simulink model "can8auto"  (R2018a)
settings: Solver=VariableStepAuto  StartTime=0.0  StopTime=5000  RelTol=1e-3
libraries: commcrc2 x20, simulink x20, simulink_extras x5, dspswit3 x5
(part 4 of 7)

== system can8auto/CAN MASTER/CAN NODE/SDO Frame generator/Subsystem/1B3 ==
  In1 : Inport
  In2 : Inport  Port=2
  In3 : Inport  Port=3
  In4 : Inport  Port=4
  Action Port : ActionPort  ActionType=case
  Mux : Mux
  Out1 : Outport
  wires:
  In4/1 -> Mux/4
  In3/1 -> Mux/3
  Mux/1 -> Out1/1
  In2/1 -> Mux/2
  In1/1 -> Mux/1

== system can8auto/CAN MASTER/CAN NODE/SDO Frame generator/Subsystem/1B4 ==
  In1 : Inport
  In2 : Inport  Port=2
  In3 : Inport  Port=3
  In4 : Inport  Port=4
  In5 : Inport  Port=5
  Action Port : ActionPort  ActionType=case
  Mux : Mux  Inputs=5
  Out1 : Outport
  wires:
  In5/1 -> Mux/5
  In4/1 -> Mux/4
  In3/1 -> Mux/3
  Mux/1 -> Out1/1
  In2/1 -> Mux/2
  In1/1 -> Mux/1

== system can8auto/CAN MASTER/CAN NODE/SDO Frame generator/Subsystem/1B5 ==
  In1 : Inport
  In2 : Inport  Port=2
  In3 : Inport  Port=3
  In4 : Inport  Port=4
  In5 : Inport  Port=5
  In6 : Inport  Port=6
  Action Port : ActionPort  ActionType=case
  Mux : Mux  Inputs=6
  Out1 : Outport
  wires:
  In6/1 -> Mux/6
  In5/1 -> Mux/5
  In4/1 -> Mux/4
  In3/1 -> Mux/3
  Mux/1 -> Out1/1
  In2/1 -> Mux/2
  In1/1 -> Mux/1

== system can8auto/CAN MASTER/CAN NODE/SDO Frame generator/Subsystem/1B6 ==
  In1 : Inport
  In2 : Inport  Port=2
  In3 : Inport  Port=3
  In4 : Inport  Port=4
  In5 : Inport  Port=5
  In6 : Inport  Port=6
  In7 : Inport  Port=7
  Action Port : ActionPort  ActionType=case
  Mux : Mux  Inputs=7
  Out1 : Outport
  wires:
  In7/1 -> Mux/7
  In6/1 -> Mux/6
  In5/1 -> Mux/5
  In4/1 -> Mux/4
  In3/1 -> Mux/3
  Mux/1 -> Out1/1
  In2/1 -> Mux/2
  In1/1 -> Mux/1

== system can8auto/CAN MASTER/CAN NODE/SDO Frame generator/Subsystem/1B7 ==
  In1 : Inport
  In2 : Inport  Port=2
  In3 : Inport  Port=3
  In4 : Inport  Port=4
  In5 : Inport  Port=5
  In6 : Inport  Port=6
  In7 : Inport  Port=7
  In8 : Inport  Port=8
  Action Port : ActionPort  ActionType=default
  Mux : Mux  Inputs=8
  Out1 : Outport
  wires:
  In8/1 -> Mux/8
  In7/1 -> Mux/7
  In6/1 -> Mux/6
  In5/1 -> Mux/5
  In4/1 -> Mux/4
  In3/1 -> Mux/3
  Mux/1 -> Out1/1
  In2/1 -> Mux/2
  In1/1 -> Mux/1

== system can8auto/CAN MASTER/CAN NODE/SDO Frame generator/Subsystem1/1B ==
  In1 : Inport
  Action Port : ActionPort  ActionType=case
  Out1 : Outport
  wires:
  In1/1 -> Out1/1

== system can8auto/CAN MASTER/CAN NODE/SDO Frame generator/Subsystem1/1B1 ==
  In1 : Inport
  In2 : Inport  Port=2
  Action Port : ActionPort  ActionType=case
  Mux : Mux  Inputs=2
  Out1 : Outport
  wires:
  Mux/1 -> Out1/1
  In2/1 -> Mux/2
  In1/1 -> Mux/1

== system can8auto/CAN MASTER/CAN NODE/SDO Frame generator/Subsystem1/1B2 ==
  In1 : Inport
  In2 : Inport  Port=2
  In3 : Inport  Port=3
  Action Port : ActionPort  ActionType=case
  Mux : Mux  Inputs=3
  Out1 : Outport
  wires:
  In3/1 -> Mux/3
  Mux/1 -> Out1/1
  In2/1 -> Mux/2
  In1/1 -> Mux/1

== system can8auto/CAN MASTER/CAN NODE/SDO Frame generator/Subsystem1/1B3 ==
  In1 : Inport
  In2 : Inport  Port=2
  In3 : Inport  Port=3
  In4 : Inport  Port=4
  Action Port : ActionPort  ActionType=case
  Mux : Mux
  Out1 : Outport
  wires:
  In4/1 -> Mux/4
  In3/1 -> Mux/3
  Mux/1 -> Out1/1
  In2/1 -> Mux/2
  In1/1 -> Mux/1

== system can8auto/CAN MASTER/CAN NODE/SDO Frame generator/Subsystem1/1B4 ==
  In1 : Inport
  In2 : Inport  Port=2
  In3 : Inport  Port=3
  In4 : Inport  Port=4
  In5 : Inport  Port=5
  Action Port : ActionPort  ActionType=case
  Mux : Mux  Inputs=5
  Out1 : Outport
  wires:
  In5/1 -> Mux/5
  In4/1 -> Mux/4
  In3/1 -> Mux/3
  Mux/1 -> Out1/1
  In2/1 -> Mux/2
  In1/1 -> Mux/1

== system can8auto/CAN MASTER/CAN NODE/SDO Frame generator/Subsystem1/1B5 ==
  In1 : Inport
  In2 : Inport  Port=2
  In3 : Inport  Port=3
  In4 : Inport  Port=4
  In5 : Inport  Port=5
  In6 : Inport  Port=6
  Action Port : ActionPort  ActionType=case
  Mux : Mux  Inputs=6
  Out1 : Outport
  wires:
  In6/1 -> Mux/6
  In5/1 -> Mux/5
  In4/1 -> Mux/4
  In3/1 -> Mux/3
  Mux/1 -> Out1/1
  In2/1 -> Mux/2
  In1/1 -> Mux/1

== system can8auto/CAN MASTER/CAN NODE/SDO Frame generator/Subsystem1/1B6 ==
  In1 : Inport
  In2 : Inport  Port=2
  In3 : Inport  Port=3
  In4 : Inport  Port=4
  In5 : Inport  Port=5
  In6 : Inport  Port=6
  In7 : Inport  Port=7
  Action Port : ActionPort  ActionType=case
  Mux : Mux  Inputs=7
  Out1 : Outport
  wires:
  In7/1 -> Mux/7
  In6/1 -> Mux/6
  In5/1 -> Mux/5
  In4/1 -> Mux/4
  In3/1 -> Mux/3
  Mux/1 -> Out1/1
  In2/1 -> Mux/2
  In1/1 -> Mux/1

== system can8auto/CAN MASTER/CAN NODE/SDO Frame generator/Subsystem1/1B7 ==
  In1 : Inport
  In2 : Inport  Port=2
  In3 : Inport  Port=3
  In4 : Inport  Port=4
  In5 : Inport  Port=5
  In6 : Inport  Port=6
  In7 : Inport  Port=7
  In8 : Inport  Port=8
  Action Port : ActionPort  ActionType=default
  Mux : Mux  Inputs=8
  Out1 : Outport
  wires:
  In8/1 -> Mux/8
  In7/1 -> Mux/7
  In6/1 -> Mux/6
  In5/1 -> Mux/5
  In4/1 -> Mux/4
  In3/1 -> Mux/3
  Mux/1 -> Out1/1
  In2/1 -> Mux/2
  In1/1 -> Mux/1

== system can8auto/CAN MASTER/CAN NODE/SDO Frame generator/Subsystem2/1B ==
  In1 : Inport
  Action Port : ActionPort  ActionType=case
  Out1 : Outport
  wires:
  In1/1 -> Out1/1

== system can8auto/CAN MASTER/CAN NODE/SDO Frame generator/Subsystem2/1B1 ==
  In1 : Inport
  In2 : Inport  Port=2
  Action Port : ActionPort  ActionType=case
  Mux : Mux  Inputs=2
  Out1 : Outport
  wires:
  Mux/1 -> Out1/1
  In2/1 -> Mux/2
  In1/1 -> Mux/1

== system can8auto/CAN MASTER/CAN NODE/SDO Frame generator/Subsystem2/1B2 ==
  In1 : Inport
  In2 : Inport  Port=2
  In3 : Inport  Port=3
  Action Port : ActionPort  ActionType=case
  Mux : Mux  Inputs=3
  Out1 : Outport
  wires:
  In3/1 -> Mux/3
  Mux/1 -> Out1/1
  In2/1 -> Mux/2
  In1/1 -> Mux/1

== system can8auto/CAN MASTER/CAN NODE/SDO Frame generator/Subsystem2/1B3 ==
  In1 : Inport
  In2 : Inport  Port=2
  In3 : Inport  Port=3
  In4 : Inport  Port=4
  Action Port : ActionPort  ActionType=case
  Mux : Mux
  Out1 : Outport
  wires:
  In4/1 -> Mux/4
  In3/1 -> Mux/3
  Mux/1 -> Out1/1
  In2/1 -> Mux/2
  In1/1 -> Mux/1

== system can8auto/CAN MASTER/CAN NODE/SDO Frame generator/Subsystem2/1B4 ==
  In1 : Inport
  In2 : Inport  Port=2
  In3 : Inport  Port=3
  In4 : Inport  Port=4
  In5 : Inport  Port=5
  Action Port : ActionPort  ActionType=case
  Mux : Mux  Inputs=5
  Out1 : Outport
  wires:
  In5/1 -> Mux/5
  In4/1 -> Mux/4
  In3/1 -> Mux/3
  Mux/1 -> Out1/1
  In2/1 -> Mux/2
  In1/1 -> Mux/1

== system can8auto/CAN MASTER/CAN NODE/SDO Frame generator/Subsystem2/1B5 ==
  In1 : Inport
  In2 : Inport  Port=2
  In3 : Inport  Port=3
  In4 : Inport  Port=4
  In5 : Inport  Port=5
  In6 : Inport  Port=6
  Action Port : ActionPort  ActionType=case
  Mux : Mux  Inputs=6
  Out1 : Outport
  wires:
  In6/1 -> Mux/6
  In5/1 -> Mux/5
  In4/1 -> Mux/4
  In3/1 -> Mux/3
  Mux/1 -> Out1/1
  In2/1 -> Mux/2
  In1/1 -> Mux/1

== system can8auto/CAN MASTER/CAN NODE/SDO Frame generator/Subsystem2/1B6 ==
  In1 : Inport
  In2 : Inport  Port=2
  In3 : Inport  Port=3
  In4 : Inport  Port=4
  In5 : Inport  Port=5
  In6 : Inport  Port=6
  In7 : Inport  Port=7
  Action Port : ActionPort  ActionType=case
  Mux : Mux  Inputs=7
  Out1 : Outport
  wires:
  In7/1 -> Mux/7
  In6/1 -> Mux/6
  In5/1 -> Mux/5
  In4/1 -> Mux/4
  In3/1 -> Mux/3
  Mux/1 -> Out1/1
  In2/1 -> Mux/2
  In1/1 -> Mux/1

== system can8auto/CAN MASTER/CAN NODE/SDO Frame generator/Subsystem2/1B7 ==
  In1 : Inport
  In2 : Inport  Port=2
  In3 : Inport  Port=3
  In4 : Inport  Port=4
  In5 : Inport  Port=5
  In6 : Inport  Port=6
  In7 : Inport  Port=7
  In8 : Inport  Port=8
  Action Port : ActionPort  ActionType=default
  Mux : Mux  Inputs=8
  Out1 : Outport
  wires:
  In8/1 -> Mux/8
  In7/1 -> Mux/7
  In6/1 -> Mux/6
  In5/1 -> Mux/5
  In4/1 -> Mux/4
  In3/1 -> Mux/3
  Mux/1 -> Out1/1
  In2/1 -> Mux/2
  In1/1 -> Mux/1

== system can8auto/CAN MASTER/CAN NODE/SDO Frame generator/Subsystem3/1B ==
  In1 : Inport
  Action Port : ActionPort  ActionType=case
  Out1 : Outport
  wires:
  In1/1 -> Out1/1

== system can8auto/CAN MASTER/CAN NODE/SDO Frame generator/Subsystem3/1B1 ==
  In1 : Inport
  In2 : Inport  Port=2
  Action Port : ActionPort  ActionType=case
  Mux : Mux  Inputs=2
  Out1 : Outport
  wires:
  Mux/1 -> Out1/1
  In2/1 -> Mux/2
  In1/1 -> Mux/1

== system can8auto/CAN MASTER/CAN NODE/SDO Frame generator/Subsystem3/1B2 ==
  In1 : Inport
  In2 : Inport  Port=2
  In3 : Inport  Port=3
  Action Port : ActionPort  ActionType=case
  Mux : Mux  Inputs=3
  Out1 : Outport
  wires:
  In3/1 -> Mux/3
  Mux/1 -> Out1/1
  In2/1 -> Mux/2
  In1/1 -> Mux/1

== system can8auto/CAN MASTER/CAN NODE/SDO Frame generator/Subsystem3/1B3 ==
  In1 : Inport
  In2 : Inport  Port=2
  In3 : Inport  Port=3
  In4 : Inport  Port=4
  Action Port : ActionPort  ActionType=case
  Mux : Mux
  Out1 : Outport
  wires:
  In4/1 -> Mux/4
  In3/1 -> Mux/3
  Mux/1 -> Out1/1
  In2/1 -> Mux/2
  In1/1 -> Mux/1

== system can8auto/CAN MASTER/CAN NODE/SDO Frame generator/Subsystem3/1B4 ==
  In1 : Inport
  In2 : Inport  Port=2
  In3 : Inport  Port=3
  In4 : Inport  Port=4
  In5 : Inport  Port=5
  Action Port : ActionPort  ActionType=case
  Mux : Mux  Inputs=5
  Out1 : Outport
  wires:
  In5/1 -> Mux/5
  In4/1 -> Mux/4
  In3/1 -> Mux/3
  Mux/1 -> Out1/1
  In2/1 -> Mux/2
  In1/1 -> Mux/1

== system can8auto/CAN MASTER/CAN NODE/SDO Frame generator/Subsystem3/1B5 ==
  In1 : Inport
  In2 : Inport  Port=2
  In3 : Inport  Port=3
  In4 : Inport  Port=4
  In5 : Inport  Port=5
  In6 : Inport  Port=6
  Action Port : ActionPort  ActionType=case
  Mux : Mux  Inputs=6
  Out1 : Outport
  wires:
  In6/1 -> Mux/6
  In5/1 -> Mux/5
  In4/1 -> Mux/4
  In3/1 -> Mux/3
  Mux/1 -> Out1/1
  In2/1 -> Mux/2
  In1/1 -> Mux/1

== system can8auto/CAN MASTER/CAN NODE/SDO Frame generator/Subsystem3/1B6 ==
  In1 : Inport
  In2 : Inport  Port=2
  In3 : Inport  Port=3
  In4 : Inport  Port=4
  In5 : Inport  Port=5
  In6 : Inport  Port=6
  In7 : Inport  Port=7
  Action Port : ActionPort  ActionType=case
  Mux : Mux  Inputs=7
  Out1 : Outport
  wires:
  In7/1 -> Mux/7
  In6/1 -> Mux/6
  In5/1 -> Mux/5
  In4/1 -> Mux/4
  In3/1 -> Mux/3
  Mux/1 -> Out1/1
  In2/1 -> Mux/2
  In1/1 -> Mux/1

== system can8auto/CAN MASTER/CAN NODE/SDO Frame generator/Subsystem3/1B7 ==
  In1 : Inport
  In2 : Inport  Port=2
  In3 : Inport  Port=3
  In4 : Inport  Port=4
  In5 : Inport  Port=5
  In6 : Inport  Port=6
  In7 : Inport  Port=7
  In8 : Inport  Port=8
  Action Port : ActionPort  ActionType=default
  Mux : Mux  Inputs=8
  Out1 : Outport
  wires:
  In8/1 -> Mux/8
  In7/1 -> Mux/7
  In6/1 -> Mux/6
  In5/1 -> Mux/5
  In4/1 -> Mux/4
  In3/1 -> Mux/3
  Mux/1 -> Out1/1
  In2/1 -> Mux/2
  In1/1 -> Mux/1

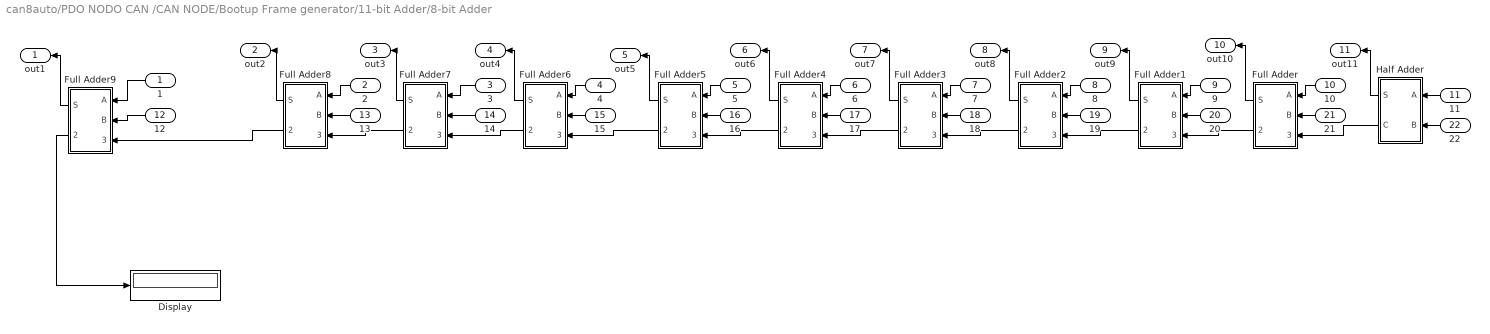
== system can8auto/PDO NODO CAN /CAN NODE/Bootup Frame generator/11-bit Adder/8-bit Adder ==
  1 : Inport
  2 : Inport  Port=2
  3 : Inport  Port=3
  4 : Inport  Port=4
  5 : Inport  Port=5
  6 : Inport  Port=6
  7 : Inport  Port=7
  8 : Inport  Port=8
  9 : Inport  Port=9
  10 : Inport  Port=10
  11 : Inport  Port=11
  12 : Inport  Port=12
  13 : Inport  Port=13
  14 : Inport  Port=14
  15 : Inport  Port=15
  16 : Inport  Port=16
  17 : Inport  Port=17
  18 : Inport  Port=18
  19 : Inport  Port=19
  20 : Inport  Port=20
  21 : Inport  Port=21
  22 : Inport  Port=22
  Display : Display
  Full Adder : Subsystem
  Full Adder1 : Subsystem
  Full Adder2 : Subsystem
  Full Adder3 : Subsystem
  Full Adder4 : Subsystem
  Full Adder5 : Subsystem
  Full Adder6 : Subsystem
  Full Adder7 : Subsystem
  Full Adder8 : Subsystem
  Full Adder9 : Subsystem
  Half Adder : Subsystem
  out1 : Outport
  out2 : Outport  Port=2
  out3 : Outport  Port=3
  out4 : Outport  Port=4
  out5 : Outport  Port=5
  out6 : Outport  Port=6
  out7 : Outport  Port=7
  out8 : Outport  Port=8
  out9 : Outport  Port=9
  out10 : Outport  Port=10
  out11 : Outport  Port=11
  wires:
  Full Adder9/2(Cout) -> Display/1
  1/1 -> Full Adder9/1(A)
  12/1 -> Full Adder9/2(B)
  13/1 -> Full Adder8/2(B)
  2/1 -> Full Adder8/1(A)
  14/1 -> Full Adder7/2(B)
  3/1 -> Full Adder7/1(A)
  Full Adder8/2(Cout) -> Full Adder9/3(Cin)
  Full Adder7/2(Cout) -> Full Adder8/3(Cin)
  Full Adder9/1(S) -> out1/1
  Full Adder8/1(S) -> out2/1
  Full Adder7/1(S) -> out3/1
  Full Adder6/2(Cout) -> Full Adder7/3(Cin)
  Half Adder/1(S) -> out11/1
  Full Adder4/1(S) -> out6/1
  Full Adder2/1(S) -> out8/1
  5/1 -> Full Adder5/1(A)
  22/1 -> Half Adder/2(B)
  Full Adder3/2(Cout) -> Full Adder4/3(Cin)
  Half Adder/2(C) -> Full Adder/3(Cin)
  Full Adder4/2(Cout) -> Full Adder5/3(Cin)
  Full Adder1/2(Cout) -> Full Adder2/3(Cin)
  Full Adder3/1(S) -> out7/1
  7/1 -> Full Adder3/1(A)
  Full Adder5/1(S) -> out5/1
  15/1 -> Full Adder6/2(B)
  19/1 -> Full Adder2/2(B)
  17/1 -> Full Adder4/2(B)
  16/1 -> Full Adder5/2(B)
  Full Adder/2(Cout) -> Full Adder1/3(Cin)
  20/1 -> Full Adder1/2(B)
  Full Adder1/1(S) -> out9/1
  6/1 -> Full Adder4/1(A)
  10/1 -> Full Adder/1(A)
  18/1 -> Full Adder3/2(B)
  4/1 -> Full Adder6/1(A)
  Full Adder6/1(S) -> out4/1
  21/1 -> Full Adder/2(B)
  Full Adder5/2(Cout) -> Full Adder6/3(Cin)
  Full Adder2/2(Cout) -> Full Adder3/3(Cin)
  11/1 -> Half Adder/1(A)
  9/1 -> Full Adder1/1(A)
  Full Adder/1(S) -> out10/1
  8/1 -> Full Adder2/1(A)

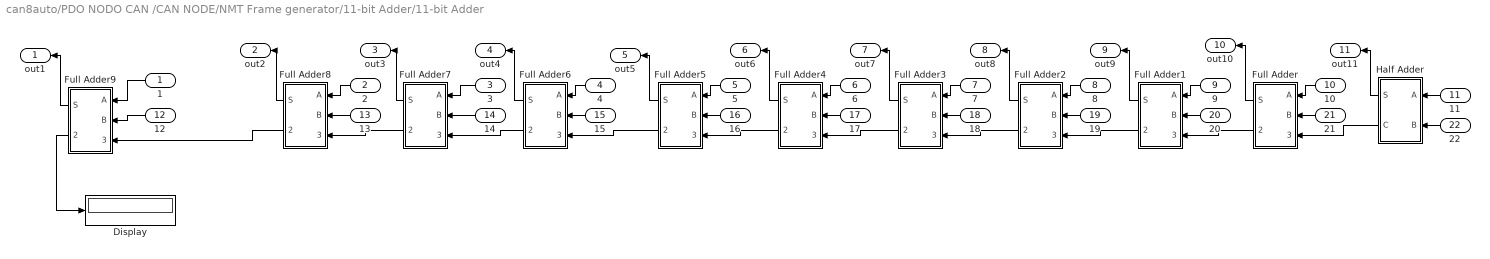
== system can8auto/PDO NODO CAN /CAN NODE/NMT Frame generator/11-bit Adder/11-bit Adder ==
  1 : Inport
  2 : Inport  Port=2
  3 : Inport  Port=3
  4 : Inport  Port=4
  5 : Inport  Port=5
  6 : Inport  Port=6
  7 : Inport  Port=7
  8 : Inport  Port=8
  9 : Inport  Port=9
  10 : Inport  Port=10
  11 : Inport  Port=11
  12 : Inport  Port=12
  13 : Inport  Port=13
  14 : Inport  Port=14
  15 : Inport  Port=15
  16 : Inport  Port=16
  17 : Inport  Port=17
  18 : Inport  Port=18
  19 : Inport  Port=19
  20 : Inport  Port=20
  21 : Inport  Port=21
  22 : Inport  Port=22
  Display : Display
  Full Adder : Subsystem
  Full Adder1 : Subsystem
  Full Adder2 : Subsystem
  Full Adder3 : Subsystem
  Full Adder4 : Subsystem
  Full Adder5 : Subsystem
  Full Adder6 : Subsystem
  Full Adder7 : Subsystem
  Full Adder8 : Subsystem
  Full Adder9 : Subsystem
  Half Adder : Subsystem
  out1 : Outport
  out2 : Outport  Port=2
  out3 : Outport  Port=3
  out4 : Outport  Port=4
  out5 : Outport  Port=5
  out6 : Outport  Port=6
  out7 : Outport  Port=7
  out8 : Outport  Port=8
  out9 : Outport  Port=9
  out10 : Outport  Port=10
  out11 : Outport  Port=11
  wires:
  Full Adder9/2(Cout) -> Display/1
  1/1 -> Full Adder9/1(A)
  12/1 -> Full Adder9/2(B)
  13/1 -> Full Adder8/2(B)
  2/1 -> Full Adder8/1(A)
  14/1 -> Full Adder7/2(B)
  3/1 -> Full Adder7/1(A)
  Full Adder8/2(Cout) -> Full Adder9/3(Cin)
  Full Adder7/2(Cout) -> Full Adder8/3(Cin)
  Full Adder9/1(S) -> out1/1
  Full Adder8/1(S) -> out2/1
  Full Adder7/1(S) -> out3/1
  Full Adder6/2(Cout) -> Full Adder7/3(Cin)
  Half Adder/1(S) -> out11/1
  Full Adder4/1(S) -> out6/1
  Full Adder2/1(S) -> out8/1
  5/1 -> Full Adder5/1(A)
  22/1 -> Half Adder/2(B)
  Full Adder3/2(Cout) -> Full Adder4/3(Cin)
  Half Adder/2(C) -> Full Adder/3(Cin)
  Full Adder4/2(Cout) -> Full Adder5/3(Cin)
  Full Adder1/2(Cout) -> Full Adder2/3(Cin)
  Full Adder3/1(S) -> out7/1
  7/1 -> Full Adder3/1(A)
  Full Adder5/1(S) -> out5/1
  15/1 -> Full Adder6/2(B)
  19/1 -> Full Adder2/2(B)
  17/1 -> Full Adder4/2(B)
  16/1 -> Full Adder5/2(B)
  Full Adder/2(Cout) -> Full Adder1/3(Cin)
  20/1 -> Full Adder1/2(B)
  Full Adder1/1(S) -> out9/1
  6/1 -> Full Adder4/1(A)
  10/1 -> Full Adder/1(A)
  18/1 -> Full Adder3/2(B)
  4/1 -> Full Adder6/1(A)
  Full Adder6/1(S) -> out4/1
  21/1 -> Full Adder/2(B)
  Full Adder5/2(Cout) -> Full Adder6/3(Cin)
  Full Adder2/2(Cout) -> Full Adder3/3(Cin)
  11/1 -> Half Adder/1(A)
  9/1 -> Full Adder1/1(A)
  Full Adder/1(S) -> out10/1
  8/1 -> Full Adder2/1(A)

== system can8auto/PDO NODO CAN /CAN NODE/PDO Frame Generator/Subsystem/1B ==
  In1 : Inport
  Action Port : ActionPort  ActionType=case
  Out1 : Outport
  wires:
  In1/1 -> Out1/1

== system can8auto/PDO NODO CAN /CAN NODE/PDO Frame Generator/Subsystem/1B1 ==
  In1 : Inport
  In2 : Inport  Port=2
  Action Port : ActionPort  ActionType=case
  Mux : Mux  Inputs=2
  Out1 : Outport
  wires:
  Mux/1 -> Out1/1
  In2/1 -> Mux/2
  In1/1 -> Mux/1

== system can8auto/PDO NODO CAN /CAN NODE/PDO Frame Generator/Subsystem/1B2 ==
  In1 : Inport
  In2 : Inport  Port=2
  In3 : Inport  Port=3
  Action Port : ActionPort  ActionType=case
  Mux : Mux  Inputs=3
  Out1 : Outport
  wires:
  In3/1 -> Mux/3
  Mux/1 -> Out1/1
  In2/1 -> Mux/2
  In1/1 -> Mux/1

== system can8auto/PDO NODO CAN /CAN NODE/PDO Frame Generator/Subsystem/1B3 ==
  In1 : Inport
  In2 : Inport  Port=2
  In3 : Inport  Port=3
  In4 : Inport  Port=4
  Action Port : ActionPort  ActionType=case
  Mux : Mux
  Out1 : Outport
  wires:
  In4/1 -> Mux/4
  In3/1 -> Mux/3
  Mux/1 -> Out1/1
  In2/1 -> Mux/2
  In1/1 -> Mux/1

== system can8auto/PDO NODO CAN /CAN NODE/PDO Frame Generator/Subsystem/1B4 ==
  In1 : Inport
  In2 : Inport  Port=2
  In3 : Inport  Port=3
  In4 : Inport  Port=4
  In5 : Inport  Port=5
  Action Port : ActionPort  ActionType=case
  Mux : Mux  Inputs=5
  Out1 : Outport
  wires:
  In5/1 -> Mux/5
  In4/1 -> Mux/4
  In3/1 -> Mux/3
  Mux/1 -> Out1/1
  In2/1 -> Mux/2
  In1/1 -> Mux/1

== system can8auto/PDO NODO CAN /CAN NODE/PDO Frame Generator/Subsystem/1B5 ==
  In1 : Inport
  In2 : Inport  Port=2
  In3 : Inport  Port=3
  In4 : Inport  Port=4
  In5 : Inport  Port=5
  In6 : Inport  Port=6
  Action Port : ActionPort  ActionType=case
  Mux : Mux  Inputs=6
  Out1 : Outport
  wires:
  In6/1 -> Mux/6
  In5/1 -> Mux/5
  In4/1 -> Mux/4
  In3/1 -> Mux/3
  Mux/1 -> Out1/1
  In2/1 -> Mux/2
  In1/1 -> Mux/1

== system can8auto/PDO NODO CAN /CAN NODE/PDO Frame Generator/Subsystem/1B6 ==
  In1 : Inport
  In2 : Inport  Port=2
  In3 : Inport  Port=3
  In4 : Inport  Port=4
  In5 : Inport  Port=5
  In6 : Inport  Port=6
  In7 : Inport  Port=7
  Action Port : ActionPort  ActionType=case
  Mux : Mux  Inputs=7
  Out1 : Outport
  wires:
  In7/1 -> Mux/7
  In6/1 -> Mux/6
  In5/1 -> Mux/5
  In4/1 -> Mux/4
  In3/1 -> Mux/3
  Mux/1 -> Out1/1
  In2/1 -> Mux/2
  In1/1 -> Mux/1

== system can8auto/PDO NODO CAN /CAN NODE/PDO Frame Generator/Subsystem/1B7 ==
  In1 : Inport
  In2 : Inport  Port=2
  In3 : Inport  Port=3
  In4 : Inport  Port=4
  In5 : Inport  Port=5
  In6 : Inport  Port=6
  In7 : Inport  Port=7
  In8 : Inport  Port=8
  Action Port : ActionPort  ActionType=default
  Mux : Mux  Inputs=8
  Out1 : Outport
  wires:
  In8/1 -> Mux/8
  In7/1 -> Mux/7
  In6/1 -> Mux/6
  In5/1 -> Mux/5
  In4/1 -> Mux/4
  In3/1 -> Mux/3
  Mux/1 -> Out1/1
  In2/1 -> Mux/2
  In1/1 -> Mux/1

== system can8auto/PDO NODO CAN /CAN NODE/SDO Frame generator/Subsystem/1B ==
  In1 : Inport
  Action Port : ActionPort  ActionType=case
  Out1 : Outport
  wires:
  In1/1 -> Out1/1

== system can8auto/PDO NODO CAN /CAN NODE/SDO Frame generator/Subsystem/1B1 ==
  In1 : Inport
  In2 : Inport  Port=2
  Action Port : ActionPort  ActionType=case
  Mux : Mux  Inputs=2
  Out1 : Outport
  wires:
  Mux/1 -> Out1/1
  In2/1 -> Mux/2
  In1/1 -> Mux/1

== system can8auto/PDO NODO CAN /CAN NODE/SDO Frame generator/Subsystem/1B2 ==
  In1 : Inport
  In2 : Inport  Port=2
  In3 : Inport  Port=3
  Action Port : ActionPort  ActionType=case
  Mux : Mux  Inputs=3
  Out1 : Outport
  wires:
  In3/1 -> Mux/3
  Mux/1 -> Out1/1
  In2/1 -> Mux/2
  In1/1 -> Mux/1

== system can8auto/PDO NODO CAN /CAN NODE/SDO Frame generator/Subsystem/1B3 ==
  In1 : Inport
  In2 : Inport  Port=2
  In3 : Inport  Port=3
  In4 : Inport  Port=4
  Action Port : ActionPort  ActionType=case
  Mux : Mux
  Out1 : Outport
  wires:
  In4/1 -> Mux/4
  In3/1 -> Mux/3
  Mux/1 -> Out1/1
  In2/1 -> Mux/2
  In1/1 -> Mux/1

== system can8auto/PDO NODO CAN /CAN NODE/SDO Frame generator/Subsystem/1B4 ==
  In1 : Inport
  In2 : Inport  Port=2
  In3 : Inport  Port=3
  In4 : Inport  Port=4
  In5 : Inport  Port=5
  Action Port : ActionPort  ActionType=case
  Mux : Mux  Inputs=5
  Out1 : Outport
  wires:
  In5/1 -> Mux/5
  In4/1 -> Mux/4
  In3/1 -> Mux/3
  Mux/1 -> Out1/1
  In2/1 -> Mux/2
  In1/1 -> Mux/1

== system can8auto/PDO NODO CAN /CAN NODE/SDO Frame generator/Subsystem/1B5 ==
  In1 : Inport
  In2 : Inport  Port=2
  In3 : Inport  Port=3
  In4 : Inport  Port=4
  In5 : Inport  Port=5
  In6 : Inport  Port=6
  Action Port : ActionPort  ActionType=case
  Mux : Mux  Inputs=6
  Out1 : Outport
  wires:
  In6/1 -> Mux/6
  In5/1 -> Mux/5
  In4/1 -> Mux/4
  In3/1 -> Mux/3
  Mux/1 -> Out1/1
  In2/1 -> Mux/2
  In1/1 -> Mux/1

== system can8auto/PDO NODO CAN /CAN NODE/SDO Frame generator/Subsystem/1B6 ==
  In1 : Inport
  In2 : Inport  Port=2
  In3 : Inport  Port=3
  In4 : Inport  Port=4
  In5 : Inport  Port=5
  In6 : Inport  Port=6
  In7 : Inport  Port=7
  Action Port : ActionPort  ActionType=case
  Mux : Mux  Inputs=7
  Out1 : Outport
  wires:
  In7/1 -> Mux/7
  In6/1 -> Mux/6
  In5/1 -> Mux/5
  In4/1 -> Mux/4
  In3/1 -> Mux/3
  Mux/1 -> Out1/1
  In2/1 -> Mux/2
  In1/1 -> Mux/1

== system can8auto/PDO NODO CAN /CAN NODE/SDO Frame generator/Subsystem/1B7 ==
  In1 : Inport
  In2 : Inport  Port=2
  In3 : Inport  Port=3
  In4 : Inport  Port=4
  In5 : Inport  Port=5
  In6 : Inport  Port=6
  In7 : Inport  Port=7
  In8 : Inport  Port=8
  Action Port : ActionPort  ActionType=default
  Mux : Mux  Inputs=8
  Out1 : Outport
  wires:
  In8/1 -> Mux/8
  In7/1 -> Mux/7
  In6/1 -> Mux/6
  In5/1 -> Mux/5
  In4/1 -> Mux/4
  In3/1 -> Mux/3
  Mux/1 -> Out1/1
  In2/1 -> Mux/2
  In1/1 -> Mux/1

== system can8auto/PDO NODO CAN /CAN NODE/SDO Frame generator/Subsystem1/1B ==
  In1 : Inport
  Action Port : ActionPort  ActionType=case
  Out1 : Outport
  wires:
  In1/1 -> Out1/1

== system can8auto/PDO NODO CAN /CAN NODE/SDO Frame generator/Subsystem1/1B1 ==
  In1 : Inport
  In2 : Inport  Port=2
  Action Port : ActionPort  ActionType=case
  Mux : Mux  Inputs=2
  Out1 : Outport
  wires:
  Mux/1 -> Out1/1
  In2/1 -> Mux/2
  In1/1 -> Mux/1

== system can8auto/PDO NODO CAN /CAN NODE/SDO Frame generator/Subsystem1/1B2 ==
  In1 : Inport
  In2 : Inport  Port=2
  In3 : Inport  Port=3
  Action Port : ActionPort  ActionType=case
  Mux : Mux  Inputs=3
  Out1 : Outport
  wires:
  In3/1 -> Mux/3
  Mux/1 -> Out1/1
  In2/1 -> Mux/2
  In1/1 -> Mux/1

== system can8auto/PDO NODO CAN /CAN NODE/SDO Frame generator/Subsystem1/1B3 ==
  In1 : Inport
  In2 : Inport  Port=2
  In3 : Inport  Port=3
  In4 : Inport  Port=4
  Action Port : ActionPort  ActionType=case
  Mux : Mux
  Out1 : Outport
  wires:
  In4/1 -> Mux/4
  In3/1 -> Mux/3
  Mux/1 -> Out1/1
  In2/1 -> Mux/2
  In1/1 -> Mux/1

== system can8auto/PDO NODO CAN /CAN NODE/SDO Frame generator/Subsystem1/1B4 ==
  In1 : Inport
  In2 : Inport  Port=2
  In3 : Inport  Port=3
  In4 : Inport  Port=4
  In5 : Inport  Port=5
  Action Port : ActionPort  ActionType=case
  Mux : Mux  Inputs=5
  Out1 : Outport
  wires:
  In5/1 -> Mux/5
  In4/1 -> Mux/4
  In3/1 -> Mux/3
  Mux/1 -> Out1/1
  In2/1 -> Mux/2
  In1/1 -> Mux/1

== system can8auto/PDO NODO CAN /CAN NODE/SDO Frame generator/Subsystem1/1B5 ==
  In1 : Inport
  In2 : Inport  Port=2
  In3 : Inport  Port=3
  In4 : Inport  Port=4
  In5 : Inport  Port=5
  In6 : Inport  Port=6
  Action Port : ActionPort  ActionType=case
  Mux : Mux  Inputs=6
  Out1 : Outport
  wires:
  In6/1 -> Mux/6
  In5/1 -> Mux/5
  In4/1 -> Mux/4
  In3/1 -> Mux/3
  Mux/1 -> Out1/1
  In2/1 -> Mux/2
  In1/1 -> Mux/1

== system can8auto/PDO NODO CAN /CAN NODE/SDO Frame generator/Subsystem1/1B6 ==
  In1 : Inport
  In2 : Inport  Port=2
  In3 : Inport  Port=3
  In4 : Inport  Port=4
  In5 : Inport  Port=5
  In6 : Inport  Port=6
  In7 : Inport  Port=7
  Action Port : ActionPort  ActionType=case
  Mux : Mux  Inputs=7
  Out1 : Outport
  wires:
  In7/1 -> Mux/7
  In6/1 -> Mux/6
  In5/1 -> Mux/5
  In4/1 -> Mux/4
  In3/1 -> Mux/3
  Mux/1 -> Out1/1
  In2/1 -> Mux/2
  In1/1 -> Mux/1

== system can8auto/PDO NODO CAN /CAN NODE/SDO Frame generator/Subsystem1/1B7 ==
  In1 : Inport
  In2 : Inport  Port=2
  In3 : Inport  Port=3
  In4 : Inport  Port=4
  In5 : Inport  Port=5
  In6 : Inport  Port=6
  In7 : Inport  Port=7
  In8 : Inport  Port=8
  Action Port : ActionPort  ActionType=default
  Mux : Mux  Inputs=8
  Out1 : Outport
  wires:
  In8/1 -> Mux/8
  In7/1 -> Mux/7
  In6/1 -> Mux/6
  In5/1 -> Mux/5
  In4/1 -> Mux/4
  In3/1 -> Mux/3
  Mux/1 -> Out1/1
  In2/1 -> Mux/2
  In1/1 -> Mux/1

== system can8auto/PDO NODO CAN /CAN NODE/SDO Frame generator/Subsystem2/1B ==
  In1 : Inport
  Action Port : ActionPort  ActionType=case
  Out1 : Outport
  wires:
  In1/1 -> Out1/1

== system can8auto/PDO NODO CAN /CAN NODE/SDO Frame generator/Subsystem2/1B1 ==
  In1 : Inport
  In2 : Inport  Port=2
  Action Port : ActionPort  ActionType=case
  Mux : Mux  Inputs=2
  Out1 : Outport
  wires:
  Mux/1 -> Out1/1
  In2/1 -> Mux/2
  In1/1 -> Mux/1

== system can8auto/PDO NODO CAN /CAN NODE/SDO Frame generator/Subsystem2/1B2 ==
  In1 : Inport
  In2 : Inport  Port=2
  In3 : Inport  Port=3
  Action Port : ActionPort  ActionType=case
  Mux : Mux  Inputs=3
  Out1 : Outport
  wires:
  In3/1 -> Mux/3
  Mux/1 -> Out1/1
  In2/1 -> Mux/2
  In1/1 -> Mux/1

== system can8auto/PDO NODO CAN /CAN NODE/SDO Frame generator/Subsystem2/1B3 ==
  In1 : Inport
  In2 : Inport  Port=2
  In3 : Inport  Port=3
  In4 : Inport  Port=4
  Action Port : ActionPort  ActionType=case
  Mux : Mux
  Out1 : Outport
  wires:
  In4/1 -> Mux/4
  In3/1 -> Mux/3
  Mux/1 -> Out1/1
  In2/1 -> Mux/2
  In1/1 -> Mux/1

== system can8auto/PDO NODO CAN /CAN NODE/SDO Frame generator/Subsystem2/1B4 ==
  In1 : Inport
  In2 : Inport  Port=2
  In3 : Inport  Port=3
  In4 : Inport  Port=4
  In5 : Inport  Port=5
  Action Port : ActionPort  ActionType=case
  Mux : Mux  Inputs=5
  Out1 : Outport
  wires:
  In5/1 -> Mux/5
  In4/1 -> Mux/4
  In3/1 -> Mux/3
  Mux/1 -> Out1/1
  In2/1 -> Mux/2
  In1/1 -> Mux/1

== system can8auto/PDO NODO CAN /CAN NODE/SDO Frame generator/Subsystem2/1B5 ==
  In1 : Inport
  In2 : Inport  Port=2
  In3 : Inport  Port=3
  In4 : Inport  Port=4
  In5 : Inport  Port=5
  In6 : Inport  Port=6
  Action Port : ActionPort  ActionType=case
  Mux : Mux  Inputs=6
  Out1 : Outport
  wires:
  In6/1 -> Mux/6
  In5/1 -> Mux/5
  In4/1 -> Mux/4
  In3/1 -> Mux/3
  Mux/1 -> Out1/1
  In2/1 -> Mux/2
  In1/1 -> Mux/1

== system can8auto/PDO NODO CAN /CAN NODE/SDO Frame generator/Subsystem2/1B6 ==
  In1 : Inport
  In2 : Inport  Port=2
  In3 : Inport  Port=3
  In4 : Inport  Port=4
  In5 : Inport  Port=5
  In6 : Inport  Port=6
  In7 : Inport  Port=7
  Action Port : ActionPort  ActionType=case
  Mux : Mux  Inputs=7
  Out1 : Outport
  wires:
  In7/1 -> Mux/7
  In6/1 -> Mux/6
  In5/1 -> Mux/5
  In4/1 -> Mux/4
  In3/1 -> Mux/3
  Mux/1 -> Out1/1
  In2/1 -> Mux/2
  In1/1 -> Mux/1

== system can8auto/PDO NODO CAN /CAN NODE/SDO Frame generator/Subsystem2/1B7 ==
  In1 : Inport
  In2 : Inport  Port=2
  In3 : Inport  Port=3
  In4 : Inport  Port=4
  In5 : Inport  Port=5
  In6 : Inport  Port=6
  In7 : Inport  Port=7
  In8 : Inport  Port=8
  Action Port : ActionPort  ActionType=default
  Mux : Mux  Inputs=8
  Out1 : Outport
  wires:
  In8/1 -> Mux/8
  In7/1 -> Mux/7
  In6/1 -> Mux/6
  In5/1 -> Mux/5
  In4/1 -> Mux/4
  In3/1 -> Mux/3
  Mux/1 -> Out1/1
  In2/1 -> Mux/2
  In1/1 -> Mux/1

== system can8auto/PDO NODO CAN /CAN NODE/SDO Frame generator/Subsystem3/1B ==
  In1 : Inport
  Action Port : ActionPort  ActionType=case
  Out1 : Outport
  wires:
  In1/1 -> Out1/1

== system can8auto/PDO NODO CAN /CAN NODE/SDO Frame generator/Subsystem3/1B1 ==
  In1 : Inport
  In2 : Inport  Port=2
  Action Port : ActionPort  ActionType=case
  Mux : Mux  Inputs=2
  Out1 : Outport
  wires:
  Mux/1 -> Out1/1
  In2/1 -> Mux/2
  In1/1 -> Mux/1

== system can8auto/PDO NODO CAN /CAN NODE/SDO Frame generator/Subsystem3/1B2 ==
  In1 : Inport
  In2 : Inport  Port=2
  In3 : Inport  Port=3
  Action Port : ActionPort  ActionType=case
  Mux : Mux  Inputs=3
  Out1 : Outport
  wires:
  In3/1 -> Mux/3
  Mux/1 -> Out1/1
  In2/1 -> Mux/2
  In1/1 -> Mux/1

== system can8auto/PDO NODO CAN /CAN NODE/SDO Frame generator/Subsystem3/1B3 ==
  In1 : Inport
  In2 : Inport  Port=2
  In3 : Inport  Port=3
  In4 : Inport  Port=4
  Action Port : ActionPort  ActionType=case
  Mux : Mux
  Out1 : Outport
  wires:
  In4/1 -> Mux/4
  In3/1 -> Mux/3
  Mux/1 -> Out1/1
  In2/1 -> Mux/2
  In1/1 -> Mux/1

== system can8auto/PDO NODO CAN /CAN NODE/SDO Frame generator/Subsystem3/1B4 ==
  In1 : Inport
  In2 : Inport  Port=2
  In3 : Inport  Port=3
  In4 : Inport  Port=4
  In5 : Inport  Port=5
  Action Port : ActionPort  ActionType=case
  Mux : Mux  Inputs=5
  Out1 : Outport
  wires:
  In5/1 -> Mux/5
  In4/1 -> Mux/4
  In3/1 -> Mux/3
  Mux/1 -> Out1/1
  In2/1 -> Mux/2
  In1/1 -> Mux/1

== system can8auto/PDO NODO CAN /CAN NODE/SDO Frame generator/Subsystem3/1B5 ==
  In1 : Inport
  In2 : Inport  Port=2
  In3 : Inport  Port=3
  In4 : Inport  Port=4
  In5 : Inport  Port=5
  In6 : Inport  Port=6
  Action Port : ActionPort  ActionType=case
  Mux : Mux  Inputs=6
  Out1 : Outport
  wires:
  In6/1 -> Mux/6
  In5/1 -> Mux/5
  In4/1 -> Mux/4
  In3/1 -> Mux/3
  Mux/1 -> Out1/1
  In2/1 -> Mux/2
  In1/1 -> Mux/1

== system can8auto/PDO NODO CAN /CAN NODE/SDO Frame generator/Subsystem3/1B6 ==
  In1 : Inport
  In2 : Inport  Port=2
  In3 : Inport  Port=3
  In4 : Inport  Port=4
  In5 : Inport  Port=5
  In6 : Inport  Port=6
  In7 : Inport  Port=7
  Action Port : ActionPort  ActionType=case
  Mux : Mux  Inputs=7
  Out1 : Outport
  wires:
  In7/1 -> Mux/7
  In6/1 -> Mux/6
  In5/1 -> Mux/5
  In4/1 -> Mux/4
  In3/1 -> Mux/3
  Mux/1 -> Out1/1
  In2/1 -> Mux/2
  In1/1 -> Mux/1

== system can8auto/PDO NODO CAN /CAN NODE/SDO Frame generator/Subsystem3/1B7 ==
  In1 : Inport
  In2 : Inport  Port=2
  In3 : Inport  Port=3
  In4 : Inport  Port=4
  In5 : Inport  Port=5
  In6 : Inport  Port=6
  In7 : Inport  Port=7
  In8 : Inport  Port=8
  Action Port : ActionPort  ActionType=default
  Mux : Mux  Inputs=8
  Out1 : Outport
  wires:
  In8/1 -> Mux/8
  In7/1 -> Mux/7
  In6/1 -> Mux/6
  In5/1 -> Mux/5
  In4/1 -> Mux/4
  In3/1 -> Mux/3
  Mux/1 -> Out1/1
  In2/1 -> Mux/2
  In1/1 -> Mux/1

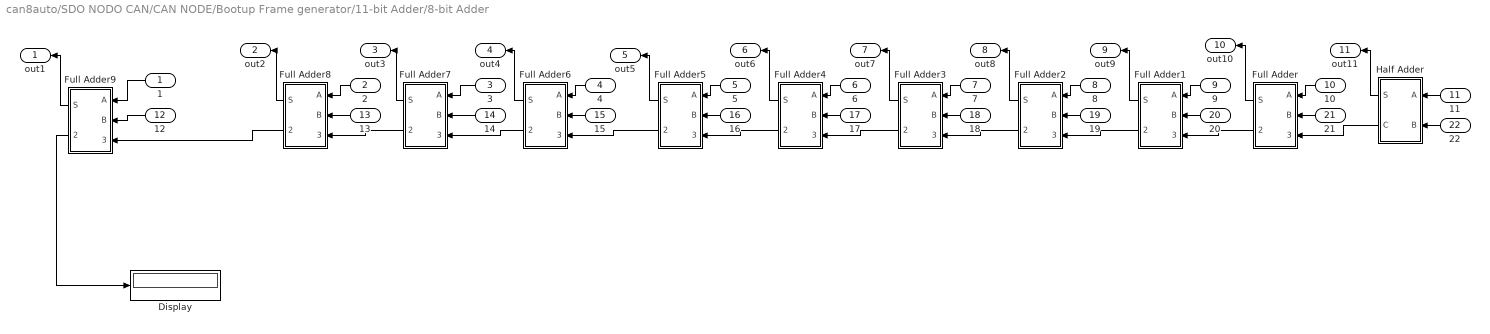
== system can8auto/SDO NODO CAN/CAN NODE/Bootup Frame generator/11-bit Adder/8-bit Adder ==
  1 : Inport
  2 : Inport  Port=2
  3 : Inport  Port=3
  4 : Inport  Port=4
  5 : Inport  Port=5
  6 : Inport  Port=6
  7 : Inport  Port=7
  8 : Inport  Port=8
  9 : Inport  Port=9
  10 : Inport  Port=10
  11 : Inport  Port=11
  12 : Inport  Port=12
  13 : Inport  Port=13
  14 : Inport  Port=14
  15 : Inport  Port=15
  16 : Inport  Port=16
  17 : Inport  Port=17
  18 : Inport  Port=18
  19 : Inport  Port=19
  20 : Inport  Port=20
  21 : Inport  Port=21
  22 : Inport  Port=22
  Display : Display
  Full Adder : Subsystem
  Full Adder1 : Subsystem
  Full Adder2 : Subsystem
  Full Adder3 : Subsystem
  Full Adder4 : Subsystem
  Full Adder5 : Subsystem
  Full Adder6 : Subsystem
  Full Adder7 : Subsystem
  Full Adder8 : Subsystem
  Full Adder9 : Subsystem
  Half Adder : Subsystem
  out1 : Outport
  out2 : Outport  Port=2
  out3 : Outport  Port=3
  out4 : Outport  Port=4
  out5 : Outport  Port=5
  out6 : Outport  Port=6
  out7 : Outport  Port=7
  out8 : Outport  Port=8
  out9 : Outport  Port=9
  out10 : Outport  Port=10
  out11 : Outport  Port=11
  wires:
  Full Adder9/2(Cout) -> Display/1
  1/1 -> Full Adder9/1(A)
  12/1 -> Full Adder9/2(B)
  13/1 -> Full Adder8/2(B)
  2/1 -> Full Adder8/1(A)
  14/1 -> Full Adder7/2(B)
  3/1 -> Full Adder7/1(A)
  Full Adder8/2(Cout) -> Full Adder9/3(Cin)
  Full Adder7/2(Cout) -> Full Adder8/3(Cin)
  Full Adder9/1(S) -> out1/1
  Full Adder8/1(S) -> out2/1
  Full Adder7/1(S) -> out3/1
  Full Adder6/2(Cout) -> Full Adder7/3(Cin)
  Half Adder/1(S) -> out11/1
  Full Adder4/1(S) -> out6/1
  Full Adder2/1(S) -> out8/1
  5/1 -> Full Adder5/1(A)
  22/1 -> Half Adder/2(B)
  Full Adder3/2(Cout) -> Full Adder4/3(Cin)
  Half Adder/2(C) -> Full Adder/3(Cin)
  Full Adder4/2(Cout) -> Full Adder5/3(Cin)
  Full Adder1/2(Cout) -> Full Adder2/3(Cin)
  Full Adder3/1(S) -> out7/1
  7/1 -> Full Adder3/1(A)
  Full Adder5/1(S) -> out5/1
  15/1 -> Full Adder6/2(B)
  19/1 -> Full Adder2/2(B)
  17/1 -> Full Adder4/2(B)
  16/1 -> Full Adder5/2(B)
  Full Adder/2(Cout) -> Full Adder1/3(Cin)
  20/1 -> Full Adder1/2(B)
  Full Adder1/1(S) -> out9/1
  6/1 -> Full Adder4/1(A)
  10/1 -> Full Adder/1(A)
  18/1 -> Full Adder3/2(B)
  4/1 -> Full Adder6/1(A)
  Full Adder6/1(S) -> out4/1
  21/1 -> Full Adder/2(B)
  Full Adder5/2(Cout) -> Full Adder6/3(Cin)
  Full Adder2/2(Cout) -> Full Adder3/3(Cin)
  11/1 -> Half Adder/1(A)
  9/1 -> Full Adder1/1(A)
  Full Adder/1(S) -> out10/1
  8/1 -> Full Adder2/1(A)

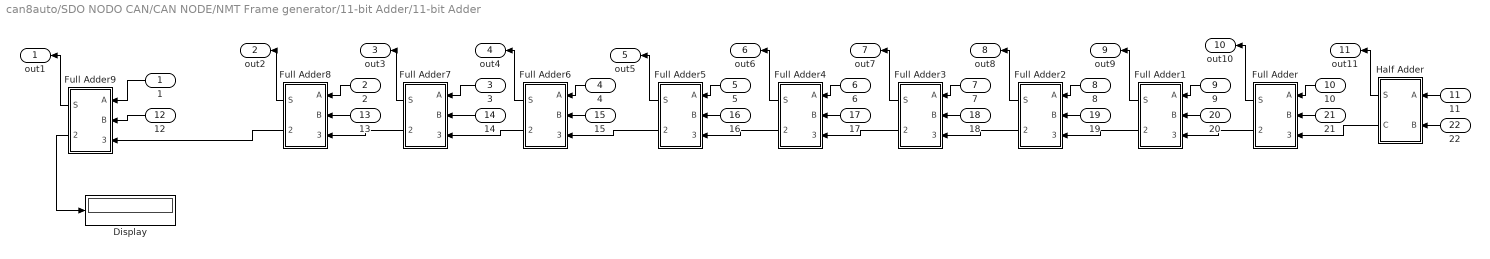
== system can8auto/SDO NODO CAN/CAN NODE/NMT Frame generator/11-bit Adder/11-bit Adder ==
  1 : Inport
  2 : Inport  Port=2
  3 : Inport  Port=3
  4 : Inport  Port=4
  5 : Inport  Port=5
  6 : Inport  Port=6
  7 : Inport  Port=7
  8 : Inport  Port=8
  9 : Inport  Port=9
  10 : Inport  Port=10
  11 : Inport  Port=11
  12 : Inport  Port=12
  13 : Inport  Port=13
  14 : Inport  Port=14
  15 : Inport  Port=15
  16 : Inport  Port=16
  17 : Inport  Port=17
  18 : Inport  Port=18
  19 : Inport  Port=19
  20 : Inport  Port=20
  21 : Inport  Port=21
  22 : Inport  Port=22
  Display : Display
  Full Adder : Subsystem
  Full Adder1 : Subsystem
  Full Adder2 : Subsystem
  Full Adder3 : Subsystem
  Full Adder4 : Subsystem
  Full Adder5 : Subsystem
  Full Adder6 : Subsystem
  Full Adder7 : Subsystem
  Full Adder8 : Subsystem
  Full Adder9 : Subsystem
  Half Adder : Subsystem
  out1 : Outport
  out2 : Outport  Port=2
  out3 : Outport  Port=3
  out4 : Outport  Port=4
  out5 : Outport  Port=5
  out6 : Outport  Port=6
  out7 : Outport  Port=7
  out8 : Outport  Port=8
  out9 : Outport  Port=9
  out10 : Outport  Port=10
  out11 : Outport  Port=11
  wires:
  Full Adder9/2(Cout) -> Display/1
  1/1 -> Full Adder9/1(A)
  12/1 -> Full Adder9/2(B)
  13/1 -> Full Adder8/2(B)
  2/1 -> Full Adder8/1(A)
  14/1 -> Full Adder7/2(B)
  3/1 -> Full Adder7/1(A)
  Full Adder8/2(Cout) -> Full Adder9/3(Cin)
  Full Adder7/2(Cout) -> Full Adder8/3(Cin)
  Full Adder9/1(S) -> out1/1
  Full Adder8/1(S) -> out2/1
  Full Adder7/1(S) -> out3/1
  Full Adder6/2(Cout) -> Full Adder7/3(Cin)
  Half Adder/1(S) -> out11/1
  Full Adder4/1(S) -> out6/1
  Full Adder2/1(S) -> out8/1
  5/1 -> Full Adder5/1(A)
  22/1 -> Half Adder/2(B)
  Full Adder3/2(Cout) -> Full Adder4/3(Cin)
  Half Adder/2(C) -> Full Adder/3(Cin)
  Full Adder4/2(Cout) -> Full Adder5/3(Cin)
  Full Adder1/2(Cout) -> Full Adder2/3(Cin)
  Full Adder3/1(S) -> out7/1
  7/1 -> Full Adder3/1(A)
  Full Adder5/1(S) -> out5/1
  15/1 -> Full Adder6/2(B)
  19/1 -> Full Adder2/2(B)
  17/1 -> Full Adder4/2(B)
  16/1 -> Full Adder5/2(B)
  Full Adder/2(Cout) -> Full Adder1/3(Cin)
  20/1 -> Full Adder1/2(B)
  Full Adder1/1(S) -> out9/1
  6/1 -> Full Adder4/1(A)
  10/1 -> Full Adder/1(A)
  18/1 -> Full Adder3/2(B)
  4/1 -> Full Adder6/1(A)
  Full Adder6/1(S) -> out4/1
  21/1 -> Full Adder/2(B)
  Full Adder5/2(Cout) -> Full Adder6/3(Cin)
  Full Adder2/2(Cout) -> Full Adder3/3(Cin)
  11/1 -> Half Adder/1(A)
  9/1 -> Full Adder1/1(A)
  Full Adder/1(S) -> out10/1
  8/1 -> Full Adder2/1(A)

== system can8auto/SDO NODO CAN/CAN NODE/PDO Frame Generator/Subsystem/1B ==
  In1 : Inport
  Action Port : ActionPort  ActionType=case
  Out1 : Outport
  wires:
  In1/1 -> Out1/1

== system can8auto/SDO NODO CAN/CAN NODE/PDO Frame Generator/Subsystem/1B1 ==
  In1 : Inport
  In2 : Inport  Port=2
  Action Port : ActionPort  ActionType=case
  Mux : Mux  Inputs=2
  Out1 : Outport
  wires:
  Mux/1 -> Out1/1
  In2/1 -> Mux/2
  In1/1 -> Mux/1

== system can8auto/SDO NODO CAN/CAN NODE/PDO Frame Generator/Subsystem/1B2 ==
  In1 : Inport
  In2 : Inport  Port=2
  In3 : Inport  Port=3
  Action Port : ActionPort  ActionType=case
  Mux : Mux  Inputs=3
  Out1 : Outport
  wires:
  In3/1 -> Mux/3
  Mux/1 -> Out1/1
  In2/1 -> Mux/2
  In1/1 -> Mux/1

== system can8auto/SDO NODO CAN/CAN NODE/PDO Frame Generator/Subsystem/1B3 ==
  In1 : Inport
  In2 : Inport  Port=2
  In3 : Inport  Port=3
  In4 : Inport  Port=4
  Action Port : ActionPort  ActionType=case
  Mux : Mux
  Out1 : Outport
  wires:
  In4/1 -> Mux/4
  In3/1 -> Mux/3
  Mux/1 -> Out1/1
  In2/1 -> Mux/2
  In1/1 -> Mux/1

== system can8auto/SDO NODO CAN/CAN NODE/PDO Frame Generator/Subsystem/1B4 ==
  In1 : Inport
  In2 : Inport  Port=2
  In3 : Inport  Port=3
  In4 : Inport  Port=4
  In5 : Inport  Port=5
  Action Port : ActionPort  ActionType=case
  Mux : Mux  Inputs=5
  Out1 : Outport
  wires:
  In5/1 -> Mux/5
  In4/1 -> Mux/4
  In3/1 -> Mux/3
  Mux/1 -> Out1/1
  In2/1 -> Mux/2
  In1/1 -> Mux/1

== system can8auto/SDO NODO CAN/CAN NODE/PDO Frame Generator/Subsystem/1B5 ==
  In1 : Inport
  In2 : Inport  Port=2
  In3 : Inport  Port=3
  In4 : Inport  Port=4
  In5 : Inport  Port=5
  In6 : Inport  Port=6
  Action Port : ActionPort  ActionType=case
  Mux : Mux  Inputs=6
  Out1 : Outport
  wires:
  In6/1 -> Mux/6
  In5/1 -> Mux/5
  In4/1 -> Mux/4
  In3/1 -> Mux/3
  Mux/1 -> Out1/1
  In2/1 -> Mux/2
  In1/1 -> Mux/1

== system can8auto/SDO NODO CAN/CAN NODE/PDO Frame Generator/Subsystem/1B6 ==
  In1 : Inport
  In2 : Inport  Port=2
  In3 : Inport  Port=3
  In4 : Inport  Port=4
  In5 : Inport  Port=5
  In6 : Inport  Port=6
  In7 : Inport  Port=7
  Action Port : ActionPort  ActionType=case
  Mux : Mux  Inputs=7
  Out1 : Outport
  wires:
  In7/1 -> Mux/7
  In6/1 -> Mux/6
  In5/1 -> Mux/5
  In4/1 -> Mux/4
  In3/1 -> Mux/3
  Mux/1 -> Out1/1
  In2/1 -> Mux/2
  In1/1 -> Mux/1

== system can8auto/SDO NODO CAN/CAN NODE/PDO Frame Generator/Subsystem/1B7 ==
  In1 : Inport
  In2 : Inport  Port=2
  In3 : Inport  Port=3
  In4 : Inport  Port=4
  In5 : Inport  Port=5
  In6 : Inport  Port=6
  In7 : Inport  Port=7
  In8 : Inport  Port=8
  Action Port : ActionPort  ActionType=default
  Mux : Mux  Inputs=8
  Out1 : Outport
  wires:
  In8/1 -> Mux/8
  In7/1 -> Mux/7
  In6/1 -> Mux/6
  In5/1 -> Mux/5
  In4/1 -> Mux/4
  In3/1 -> Mux/3
  Mux/1 -> Out1/1
  In2/1 -> Mux/2
  In1/1 -> Mux/1

== system can8auto/SDO NODO CAN/CAN NODE/SDO Frame generator/Subsystem/1B ==
  In1 : Inport
  Action Port : ActionPort  ActionType=case
  Out1 : Outport
  wires:
  In1/1 -> Out1/1

== system can8auto/SDO NODO CAN/CAN NODE/SDO Frame generator/Subsystem/1B1 ==
  In1 : Inport
  In2 : Inport  Port=2
  Action Port : ActionPort  ActionType=case
  Mux : Mux  Inputs=2
  Out1 : Outport
  wires:
  Mux/1 -> Out1/1
  In2/1 -> Mux/2
  In1/1 -> Mux/1

== system can8auto/SDO NODO CAN/CAN NODE/SDO Frame generator/Subsystem/1B2 ==
  In1 : Inport
  In2 : Inport  Port=2
  In3 : Inport  Port=3
  Action Port : ActionPort  ActionType=case
  Mux : Mux  Inputs=3
  Out1 : Outport
  wires:
  In3/1 -> Mux/3
  Mux/1 -> Out1/1
  In2/1 -> Mux/2
  In1/1 -> Mux/1

== system can8auto/SDO NODO CAN/CAN NODE/SDO Frame generator/Subsystem/1B3 ==
  In1 : Inport
  In2 : Inport  Port=2
  In3 : Inport  Port=3
  In4 : Inport  Port=4
  Action Port : ActionPort  ActionType=case
  Mux : Mux
  Out1 : Outport
  wires:
  In4/1 -> Mux/4
  In3/1 -> Mux/3
  Mux/1 -> Out1/1
  In2/1 -> Mux/2
  In1/1 -> Mux/1

== system can8auto/SDO NODO CAN/CAN NODE/SDO Frame generator/Subsystem/1B4 ==
  In1 : Inport
  In2 : Inport  Port=2
  In3 : Inport  Port=3
  In4 : Inport  Port=4
  In5 : Inport  Port=5
  Action Port : ActionPort  ActionType=case
  Mux : Mux  Inputs=5
  Out1 : Outport
  wires:
  In5/1 -> Mux/5
  In4/1 -> Mux/4
  In3/1 -> Mux/3
  Mux/1 -> Out1/1
  In2/1 -> Mux/2
  In1/1 -> Mux/1

== system can8auto/SDO NODO CAN/CAN NODE/SDO Frame generator/Subsystem/1B5 ==
  In1 : Inport
  In2 : Inport  Port=2
  In3 : Inport  Port=3
  In4 : Inport  Port=4
  In5 : Inport  Port=5
  In6 : Inport  Port=6
  Action Port : ActionPort  ActionType=case
  Mux : Mux  Inputs=6
  Out1 : Outport
  wires:
  In6/1 -> Mux/6
  In5/1 -> Mux/5
  In4/1 -> Mux/4
  In3/1 -> Mux/3
  Mux/1 -> Out1/1
  In2/1 -> Mux/2
  In1/1 -> Mux/1

== system can8auto/SDO NODO CAN/CAN NODE/SDO Frame generator/Subsystem/1B6 ==
  In1 : Inport
  In2 : Inport  Port=2
  In3 : Inport  Port=3
  In4 : Inport  Port=4
  In5 : Inport  Port=5
  In6 : Inport  Port=6
  In7 : Inport  Port=7
  Action Port : ActionPort  ActionType=case
  Mux : Mux  Inputs=7
  Out1 : Outport
  wires:
  In7/1 -> Mux/7
  In6/1 -> Mux/6
  In5/1 -> Mux/5
  In4/1 -> Mux/4
  In3/1 -> Mux/3
  Mux/1 -> Out1/1
  In2/1 -> Mux/2
  In1/1 -> Mux/1

== system can8auto/SDO NODO CAN/CAN NODE/SDO Frame generator/Subsystem/1B7 ==
  In1 : Inport
  In2 : Inport  Port=2
  In3 : Inport  Port=3
  In4 : Inport  Port=4
  In5 : Inport  Port=5
  In6 : Inport  Port=6
  In7 : Inport  Port=7
  In8 : Inport  Port=8
  Action Port : ActionPort  ActionType=default
  Mux : Mux  Inputs=8
  Out1 : Outport
  wires:
  In8/1 -> Mux/8
  In7/1 -> Mux/7
  In6/1 -> Mux/6
  In5/1 -> Mux/5
  In4/1 -> Mux/4
  In3/1 -> Mux/3
  Mux/1 -> Out1/1
  In2/1 -> Mux/2
  In1/1 -> Mux/1

== system can8auto/SDO NODO CAN/CAN NODE/SDO Frame generator/Subsystem1/1B ==
  In1 : Inport
  Action Port : ActionPort  ActionType=case
  Out1 : Outport
  wires:
  In1/1 -> Out1/1

== system can8auto/SDO NODO CAN/CAN NODE/SDO Frame generator/Subsystem1/1B1 ==
  In1 : Inport
  In2 : Inport  Port=2
  Action Port : ActionPort  ActionType=case
  Mux : Mux  Inputs=2
  Out1 : Outport
  wires:
  Mux/1 -> Out1/1
  In2/1 -> Mux/2
  In1/1 -> Mux/1

== system can8auto/SDO NODO CAN/CAN NODE/SDO Frame generator/Subsystem1/1B2 ==
  In1 : Inport
  In2 : Inport  Port=2
  In3 : Inport  Port=3
  Action Port : ActionPort  ActionType=case
  Mux : Mux  Inputs=3
  Out1 : Outport
  wires:
  In3/1 -> Mux/3
  Mux/1 -> Out1/1
  In2/1 -> Mux/2
  In1/1 -> Mux/1

== system can8auto/SDO NODO CAN/CAN NODE/SDO Frame generator/Subsystem1/1B3 ==
  In1 : Inport
  In2 : Inport  Port=2
  In3 : Inport  Port=3
  In4 : Inport  Port=4
  Action Port : ActionPort  ActionType=case
  Mux : Mux
  Out1 : Outport
  wires:
  In4/1 -> Mux/4
  In3/1 -> Mux/3
  Mux/1 -> Out1/1
  In2/1 -> Mux/2
  In1/1 -> Mux/1

== system can8auto/SDO NODO CAN/CAN NODE/SDO Frame generator/Subsystem1/1B4 ==
  In1 : Inport
  In2 : Inport  Port=2
  In3 : Inport  Port=3
  In4 : Inport  Port=4
  In5 : Inport  Port=5
  Action Port : ActionPort  ActionType=case
  Mux : Mux  Inputs=5
  Out1 : Outport
  wires:
  In5/1 -> Mux/5
  In4/1 -> Mux/4
  In3/1 -> Mux/3
  Mux/1 -> Out1/1
  In2/1 -> Mux/2
  In1/1 -> Mux/1

== system can8auto/SDO NODO CAN/CAN NODE/SDO Frame generator/Subsystem1/1B5 ==
  In1 : Inport
  In2 : Inport  Port=2
  In3 : Inport  Port=3
  In4 : Inport  Port=4
  In5 : Inport  Port=5
  In6 : Inport  Port=6
  Action Port : ActionPort  ActionType=case
  Mux : Mux  Inputs=6
  Out1 : Outport
  wires:
  In6/1 -> Mux/6
  In5/1 -> Mux/5
  In4/1 -> Mux/4
  In3/1 -> Mux/3
  Mux/1 -> Out1/1
  In2/1 -> Mux/2
  In1/1 -> Mux/1

== system can8auto/SDO NODO CAN/CAN NODE/SDO Frame generator/Subsystem1/1B6 ==
  In1 : Inport
  In2 : Inport  Port=2
  In3 : Inport  Port=3
  In4 : Inport  Port=4
  In5 : Inport  Port=5
  In6 : Inport  Port=6
  In7 : Inport  Port=7
  Action Port : ActionPort  ActionType=case
  Mux : Mux  Inputs=7
  Out1 : Outport
  wires:
  In7/1 -> Mux/7
  In6/1 -> Mux/6
  In5/1 -> Mux/5
  In4/1 -> Mux/4
  In3/1 -> Mux/3
  Mux/1 -> Out1/1
  In2/1 -> Mux/2
  In1/1 -> Mux/1

== system can8auto/SDO NODO CAN/CAN NODE/SDO Frame generator/Subsystem1/1B7 ==
  In1 : Inport
  In2 : Inport  Port=2
  In3 : Inport  Port=3
  In4 : Inport  Port=4
  In5 : Inport  Port=5
  In6 : Inport  Port=6
  In7 : Inport  Port=7
  In8 : Inport  Port=8
  Action Port : ActionPort  ActionType=default
  Mux : Mux  Inputs=8
  Out1 : Outport
  wires:
  In8/1 -> Mux/8
  In7/1 -> Mux/7
  In6/1 -> Mux/6
  In5/1 -> Mux/5
  In4/1 -> Mux/4
  In3/1 -> Mux/3
  Mux/1 -> Out1/1
  In2/1 -> Mux/2
  In1/1 -> Mux/1

== system can8auto/SDO NODO CAN/CAN NODE/SDO Frame generator/Subsystem2/1B ==
  In1 : Inport
  Action Port : ActionPort  ActionType=case
  Out1 : Outport
  wires:
  In1/1 -> Out1/1

== system can8auto/SDO NODO CAN/CAN NODE/SDO Frame generator/Subsystem2/1B1 ==
  In1 : Inport
  In2 : Inport  Port=2
  Action Port : ActionPort  ActionType=case
  Mux : Mux  Inputs=2
  Out1 : Outport
  wires:
  Mux/1 -> Out1/1
  In2/1 -> Mux/2
  In1/1 -> Mux/1

== system can8auto/SDO NODO CAN/CAN NODE/SDO Frame generator/Subsystem2/1B2 ==
  In1 : Inport
  In2 : Inport  Port=2
  In3 : Inport  Port=3
  Action Port : ActionPort  ActionType=case
  Mux : Mux  Inputs=3
  Out1 : Outport
  wires:
  In3/1 -> Mux/3
  Mux/1 -> Out1/1
  In2/1 -> Mux/2
  In1/1 -> Mux/1

== system can8auto/SDO NODO CAN/CAN NODE/SDO Frame generator/Subsystem2/1B3 ==
  In1 : Inport
  In2 : Inport  Port=2
  In3 : Inport  Port=3
  In4 : Inport  Port=4
  Action Port : ActionPort  ActionType=case
  Mux : Mux
  Out1 : Outport
  wires:
  In4/1 -> Mux/4
  In3/1 -> Mux/3
  Mux/1 -> Out1/1
  In2/1 -> Mux/2
  In1/1 -> Mux/1

== system can8auto/SDO NODO CAN/CAN NODE/SDO Frame generator/Subsystem2/1B4 ==
  In1 : Inport
  In2 : Inport  Port=2
  In3 : Inport  Port=3
  In4 : Inport  Port=4
  In5 : Inport  Port=5
  Action Port : ActionPort  ActionType=case
  Mux : Mux  Inputs=5
  Out1 : Outport
  wires:
  In5/1 -> Mux/5
  In4/1 -> Mux/4
  In3/1 -> Mux/3
  Mux/1 -> Out1/1
  In2/1 -> Mux/2
  In1/1 -> Mux/1

== system can8auto/SDO NODO CAN/CAN NODE/SDO Frame generator/Subsystem2/1B5 ==
  In1 : Inport
  In2 : Inport  Port=2
  In3 : Inport  Port=3
  In4 : Inport  Port=4
  In5 : Inport  Port=5
  In6 : Inport  Port=6
  Action Port : ActionPort  ActionType=case
  Mux : Mux  Inputs=6
  Out1 : Outport
  wires:
  In6/1 -> Mux/6
  In5/1 -> Mux/5
  In4/1 -> Mux/4
  In3/1 -> Mux/3
  Mux/1 -> Out1/1
  In2/1 -> Mux/2
  In1/1 -> Mux/1

== system can8auto/SDO NODO CAN/CAN NODE/SDO Frame generator/Subsystem2/1B6 ==
  In1 : Inport
  In2 : Inport  Port=2
  In3 : Inport  Port=3
  In4 : Inport  Port=4
  In5 : Inport  Port=5
  In6 : Inport  Port=6
  In7 : Inport  Port=7
  Action Port : ActionPort  ActionType=case
  Mux : Mux  Inputs=7
  Out1 : Outport
  wires:
  In7/1 -> Mux/7
  In6/1 -> Mux/6
  In5/1 -> Mux/5
  In4/1 -> Mux/4
  In3/1 -> Mux/3
  Mux/1 -> Out1/1
  In2/1 -> Mux/2
  In1/1 -> Mux/1

== system can8auto/SDO NODO CAN/CAN NODE/SDO Frame generator/Subsystem2/1B7 ==
  In1 : Inport
  In2 : Inport  Port=2
  In3 : Inport  Port=3
  In4 : Inport  Port=4
  In5 : Inport  Port=5
  In6 : Inport  Port=6
  In7 : Inport  Port=7
  In8 : Inport  Port=8
  Action Port : ActionPort  ActionType=default
  Mux : Mux  Inputs=8
  Out1 : Outport
  wires:
  In8/1 -> Mux/8
  In7/1 -> Mux/7
  In6/1 -> Mux/6
  In5/1 -> Mux/5
  In4/1 -> Mux/4
  In3/1 -> Mux/3
  Mux/1 -> Out1/1
  In2/1 -> Mux/2
  In1/1 -> Mux/1

== system can8auto/SDO NODO CAN/CAN NODE/SDO Frame generator/Subsystem3/1B ==
  In1 : Inport
  Action Port : ActionPort  ActionType=case
  Out1 : Outport
  wires:
  In1/1 -> Out1/1

== system can8auto/SDO NODO CAN/CAN NODE/SDO Frame generator/Subsystem3/1B1 ==
  In1 : Inport
  In2 : Inport  Port=2
  Action Port : ActionPort  ActionType=case
  Mux : Mux  Inputs=2
  Out1 : Outport
  wires:
  Mux/1 -> Out1/1
  In2/1 -> Mux/2
  In1/1 -> Mux/1

== system can8auto/SDO NODO CAN/CAN NODE/SDO Frame generator/Subsystem3/1B2 ==
  In1 : Inport
  In2 : Inport  Port=2
  In3 : Inport  Port=3
  Action Port : ActionPort  ActionType=case
  Mux : Mux  Inputs=3
  Out1 : Outport
  wires:
  In3/1 -> Mux/3
  Mux/1 -> Out1/1
  In2/1 -> Mux/2
  In1/1 -> Mux/1

== system can8auto/SDO NODO CAN/CAN NODE/SDO Frame generator/Subsystem3/1B3 ==
  In1 : Inport
  In2 : Inport  Port=2
  In3 : Inport  Port=3
  In4 : Inport  Port=4
  Action Port : ActionPort  ActionType=case
  Mux : Mux
  Out1 : Outport
  wires:
  In4/1 -> Mux/4
  In3/1 -> Mux/3
  Mux/1 -> Out1/1
  In2/1 -> Mux/2
  In1/1 -> Mux/1

== system can8auto/SDO NODO CAN/CAN NODE/SDO Frame generator/Subsystem3/1B4 ==
  In1 : Inport
  In2 : Inport  Port=2
  In3 : Inport  Port=3
  In4 : Inport  Port=4
  In5 : Inport  Port=5
  Action Port : ActionPort  ActionType=case
  Mux : Mux  Inputs=5
  Out1 : Outport
  wires:
  In5/1 -> Mux/5
  In4/1 -> Mux/4
  In3/1 -> Mux/3
  Mux/1 -> Out1/1
  In2/1 -> Mux/2
  In1/1 -> Mux/1

== system can8auto/SDO NODO CAN/CAN NODE/SDO Frame generator/Subsystem3/1B5 ==
  In1 : Inport
  In2 : Inport  Port=2
  In3 : Inport  Port=3
  In4 : Inport  Port=4
  In5 : Inport  Port=5
  In6 : Inport  Port=6
  Action Port : ActionPort  ActionType=case
  Mux : Mux  Inputs=6
  Out1 : Outport
  wires:
  In6/1 -> Mux/6
  In5/1 -> Mux/5
  In4/1 -> Mux/4
  In3/1 -> Mux/3
  Mux/1 -> Out1/1
  In2/1 -> Mux/2
  In1/1 -> Mux/1

== system can8auto/SDO NODO CAN/CAN NODE/SDO Frame generator/Subsystem3/1B6 ==
  In1 : Inport
  In2 : Inport  Port=2
  In3 : Inport  Port=3
  In4 : Inport  Port=4
  In5 : Inport  Port=5
  In6 : Inport  Port=6
  In7 : Inport  Port=7
  Action Port : ActionPort  ActionType=case
  Mux : Mux  Inputs=7
  Out1 : Outport
  wires:
  In7/1 -> Mux/7
  In6/1 -> Mux/6
  In5/1 -> Mux/5
  In4/1 -> Mux/4
  In3/1 -> Mux/3
  Mux/1 -> Out1/1
  In2/1 -> Mux/2
  In1/1 -> Mux/1

== system can8auto/SDO NODO CAN/CAN NODE/SDO Frame generator/Subsystem3/1B7 ==
  In1 : Inport
  In2 : Inport  Port=2
  In3 : Inport  Port=3
  In4 : Inport  Port=4
  In5 : Inport  Port=5
  In6 : Inport  Port=6
  In7 : Inport  Port=7
  In8 : Inport  Port=8
  Action Port : ActionPort  ActionType=default
  Mux : Mux  Inputs=8
  Out1 : Outport
  wires:
  In8/1 -> Mux/8
  In7/1 -> Mux/7
  In6/1 -> Mux/6
  In5/1 -> Mux/5
  In4/1 -> Mux/4
  In3/1 -> Mux/3
  Mux/1 -> Out1/1
  In2/1 -> Mux/2
  In1/1 -> Mux/1
